simulink model "desatsim"  (R2018a)
settings: Solver=FixedStepAuto  StartTime=0.0  StopTime=10000  FixedStep=10  RelTol=1e-3
values from neighbouring files (symbols this model uses):
  h_orbit_eci = h_orbit_ecis(1:3,i)    [desattest.m]
  hCom_sat_eci = hCom_sat_ecis(1:3,i)    [desattest.m]
  HMAG = 0.00675    [desattest.m]
  ri_orbit_eci = ri_orbit_ecis(1:3,i)    [desattest.m]
undefined symbols (not defined in the file or in its folder): Earth, IAU, init, WGS84
libraries: aerolibtransform2 x3, sharedutil x2, dspmathops x1, aerolibgravity2 x1
settings Model: Creator=nathan  LastModifiedBy=nathan

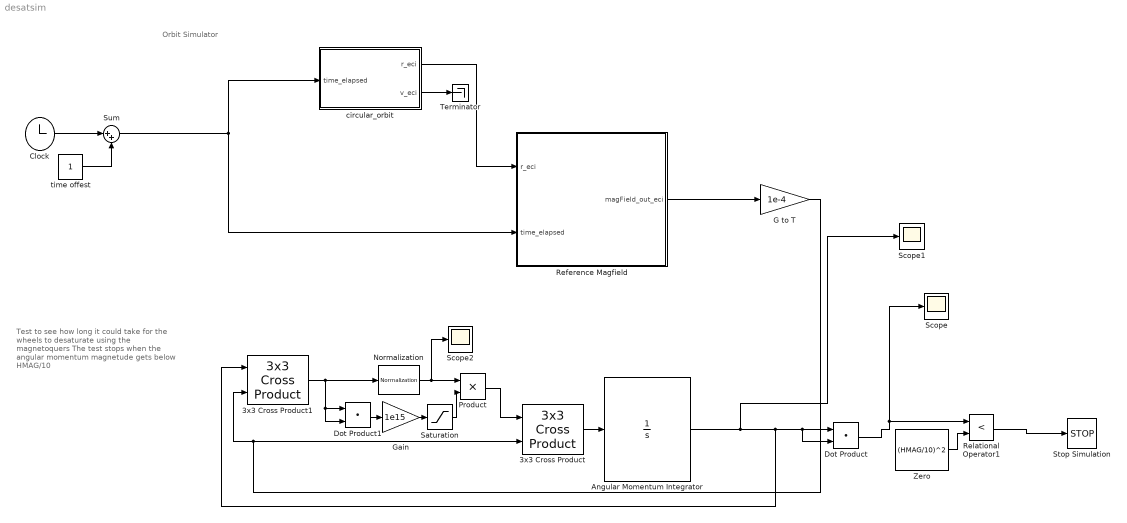
== system desatsim ==
  note: Test to see how long it could take for the wheels to desaturate using the magnetoquers
      |
      | The test stops when the angular momentum magnetude gets below HMAG/10
  note: Orbit Simulator
  3x3 Cross Product : sharedutil/3x3 Cross Product  aMode=aMode
      settings: SourceProductBaseCode=AE
  3x3 Cross Product1 : sharedutil/3x3 Cross Product  aMode=aMode
      settings: SourceProductBaseCode=AE
  Angular Momentum Integrator : Integrator  InitialCondition=hCom_sat_eci
  Clock : Clock
  Dot Product : DotProduct  InputSameDT=on  OutDataTypeStr=Inherit: Inherit via internal rule
  Dot Product1 : DotProduct  InputSameDT=on  OutDataTypeStr=Inherit: Inherit via internal rule
  G to T : Gain  Gain=1e-4
  Gain : Gain  Gain=1e15
  Normalization : dspmathops/Normalization  NormType=2-norm  Bias=1e-30  NormOver=Each column  Dimension=1  roundingMode=Floor  overflowMode=off  accumDataTypeStr=Inherit: Same as product output  accumLastDataTypeStr=Inherit: Same as product output  outputDataTypeStr=Inherit: Same as product output  outputMin=[]  outputMax=[]  outputLastDataTypeStr=Inherit: Same as product output
      settings: SourceProductName=DSP System Toolbox
  Product : Product
  "Reference Magfield " : Subsystem
  Relational Operator1 : RelationalOperator  Operator=<  OutDataTypeStr=boolean  RndMeth=Simplest
  Saturation : Saturate  UpperLimit=0.08  LowerLimit=0
  Scope : Scope
  Scope1 : Scope
  Scope2 : Scope
  Stop Simulation : Stop
  Sum : Sum  Inputs=|++
  Terminator : Terminator
  Zero : Constant  Value=(HMAG/10)^2
  circular_orbit : Subsystem  mask{P=ri_orbit_eci, H=h_orbit_eci}
      mask prompts: P "initial position in ECI, units m."; H "angular momuntum/mass in ECI units m^2/s"
      mask init:
      | W= norm(H)/dot(P,P); 
      | %angular rate magnitude, units rad/s
      | PPERP= cross(H,P)/norm(H); 
      | %position in orbit pi/2 phase shifted to the right from P, in ECI units m
      mask DialogControl DescTextVar Prompt: Circular Orbit Propagator
  time offest : Constant
  wires:
  circular_orbit/1(r_eci) -> "Reference Magfield "/1(r_eci)
  3x3 Cross Product/1 -> Angular Momentum Integrator/1
  Angular Momentum Integrator/1 -> Scope1/1, Dot Product/2, Dot Product/1, 3x3 Cross Product1/1
  3x3 Cross Product1/1 -> Normalization/1, Dot Product1/2, Dot Product1/1
  Normalization/1 -> Product/1, Scope2/1
  Product/1 -> 3x3 Cross Product/1
  Dot Product/1 -> Relational Operator1/1, Scope/1
  "Reference Magfield "/1(magField_out_eci) -> G to T/1
  G to T/1 -> 3x3 Cross Product/2, 3x3 Cross Product1/2
  Clock/1 -> Sum/1
  time offest/1 -> Sum/2
  Sum/1 -> "Reference Magfield "/2(time_elapsed), circular_orbit/1(time_elapsed)
  circular_orbit/2(v_eci) -> Terminator/1
  Zero/1 -> Relational Operator1/2
  Relational Operator1/1 -> Stop Simulation/1
  Saturation/1 -> Product/2
  Dot Product1/1 -> Gain/1
  Gain/1 -> Saturation/1

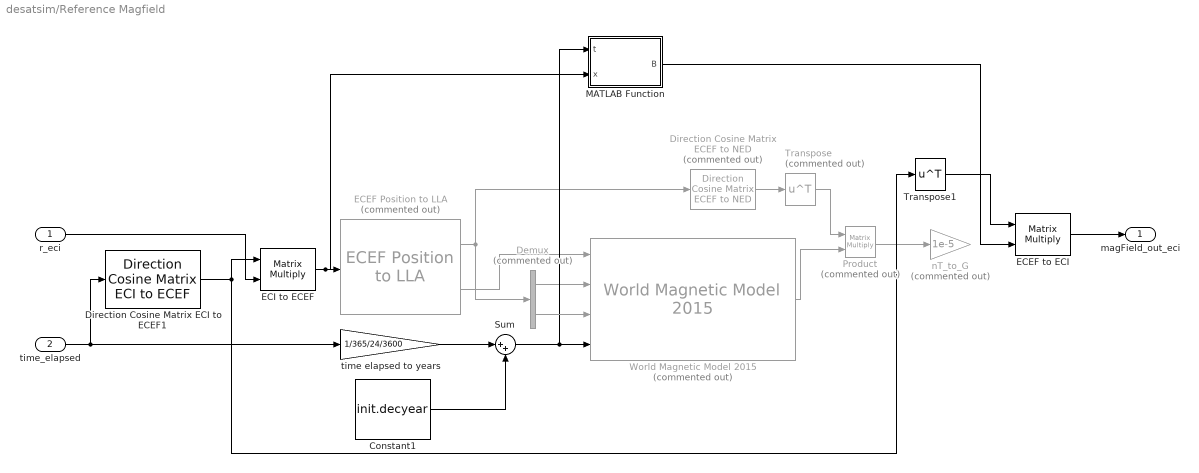
== system desatsim/Reference Magfield  ==
  r_eci : Inport  Unit=m  PortDimensions=3
  time_elapsed : Inport  Port=2  Unit=s  PortDimensions=1
  Constant1 : Constant  Value=init.decyear
  Demux : Demux  Commented=on  Outputs=2
  Direction Cosine Matrix ECEF to NED : aerolibtransform2/Direction Cosine Matrix ECEF to NED  Commented=on
      settings: SourceProductName=Aerospace Blockset  SourceProductBaseCode=AE
  Direction Cosine Matrix ECI to ECEF1 : aerolibtransform2/Direction Cosine Matrix ECI to ECEF  red=IAU-2000/2006  year=init.year  month=October  day=20  hour=init.hour  min=init.min  sec=init.sec  deltaT=Sec  errorflag=Error  extraparamflag=off
      settings: AttributesFormatString=%<red>  SourceProductName=Aerospace Blockset  SourceProductBaseCode=AE
  ECEF Position to LLA : aerolibtransform2/ECEF Position to LLA  Commented=on  units=Metric (MKS)  ptype=Earth (WGS84)  F=1/298.257223563  R=6378137
      settings: SourceProductName=Aerospace Blockset  SourceProductBaseCode=AE
  ECEF to ECI : Product  Multiplication=Matrix(*)  OutDataTypeStr=double
  ECI to ECEF : Product  Multiplication=Matrix(*)  OutDataTypeStr=double
  MATLAB Function : MATLAB Function  TreatAsAtomicUnit=on
  Product : Product  Commented=on  Multiplication=Matrix(*)
  Sum : Sum  Inputs=|++
  Transpose : Math  Commented=on  Operator=transpose  SaturateOnIntegerOverflow=on
  Transpose1 : Math  Operator=transpose  SaturateOnIntegerOverflow=on
  World Magnetic Model 2015 : aerolibgravity2/World Magnetic Model 2015  Commented=on  units=Metric (MKS)  time_in=on  month=January  day=1  year=2015  action=None  h_out=off  dec_out=off  inc_out=off  ti_out=off
      settings: SourceProductName=Aerospace Blockset  SourceProductBaseCode=AE
  nT_to_G : Gain  Commented=on  Gain=1e-5
  time elapsed to years : Gain  Gain=1/365/24/3600
  magField_out_eci : Outport  Unit=G  PortDimensions=3
  wires:
  ECEF Position to LLA/1 -> Demux/1, Direction Cosine Matrix ECEF to NED/1
  Direction Cosine Matrix ECEF to NED/1 -> Transpose/1
  Transpose/1 -> Product/1
  World Magnetic Model 2015/1 -> Product/2
  Product/1 -> nT_to_G/1
  Demux/1 -> World Magnetic Model 2015/2
  ECEF Position to LLA/2 -> World Magnetic Model 2015/1
  Sum/1 -> MATLAB Function/1(t), World Magnetic Model 2015/4
  Demux/2 -> World Magnetic Model 2015/3
  time elapsed to years/1 -> Sum/1
  Constant1/1 -> Sum/2
  time_elapsed/1 -> time elapsed to years/1, Direction Cosine Matrix ECI to ECEF1/1
  Direction Cosine Matrix ECI to ECEF1/1 -> Transpose1/1, ECI to ECEF/1
  r_eci/1 -> ECI to ECEF/2
  ECI to ECEF/1 -> MATLAB Function/2(x), ECEF Position to LLA/1
  Transpose1/1 -> ECEF to ECI/1
  ECEF to ECI/1 -> magField_out_eci/1
  MATLAB Function/1(B) -> ECEF to ECI/2

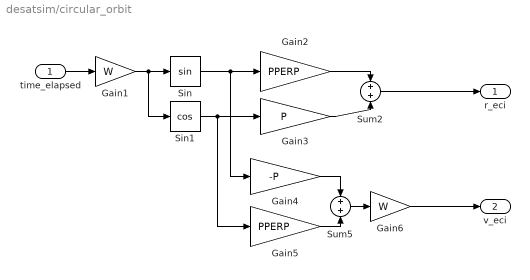
== system desatsim/circular_orbit ==
  time_elapsed : Inport  Unit=s  PortDimensions=1
  Gain1 : Gain  Gain=W
  Gain2 : Gain  Gain=PPERP
  Gain3 : Gain  Gain=P
  Gain4 : Gain  Gain=-P
  Gain5 : Gain  Gain=PPERP
  Gain6 : Gain  Gain=W
  Sin : Trigonometry
  Sin1 : Trigonometry  Operator=cos
  Sum2 : Sum  Inputs=+|+
  Sum5 : Sum  Inputs=+|+
  r_eci : Outport  Unit=m  PortDimensions=3
  v_eci : Outport  Port=2  Unit=m/s  PortDimensions=3
  wires:
  Gain5/1 -> Sum5/2
  Sum2/1 -> r_eci/1
  Gain2/1 -> Sum2/1
  Gain3/1 -> Sum2/2
  Gain4/1 -> Sum5/1
  Gain1/1 -> Sin/1, Sin1/1
  Sin1/1 -> Gain5/1, Gain3/1
  time_elapsed/1 -> Gain1/1
  Sum5/1 -> Gain6/1
  Sin/1 -> Gain4/1, Gain2/1
  Gain6/1 -> v_eci/1

== matlab function desatsim/Reference Magfield /MATLAB Function ==
  data: t input; B output; x input
function B = fcn(t,x)
%sds
B= refMag(t,x);
